simulink model "msiglabel_in"  (Simulink 6.3)
settings: Solver=FixedStepDiscrete  StartTime=0.0  StopTime=10.0  RelTol=1e-3
settings Model: Creator=awarlock  LastModifiedBy=mshakeri  ExtModeAutoUpdateStatusClock=off  StrictBusMsg=ErrorLevel1
settings OptimizationCC: InlineParams=on  InlineInvariantSignals=on
settings DebuggingCC: CheckExecutionContextPreStartOutputMsg=on  CheckExecutionContextRuntimeOutputMsg=on  SolverPrmCheckMsg=none  UnconnectedInputMsg=none  UnconnectedOutputMsg=none  UnconnectedLineMsg=none

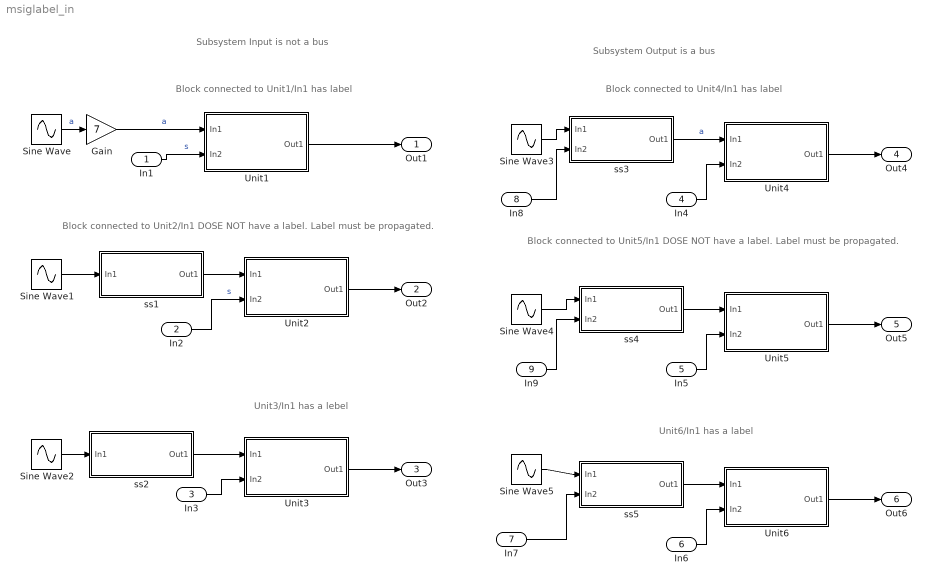
== system msiglabel_in ==
  note: Block connected to Unit1/In1 has label
  note: Block connected to Unit2/In1 DOSE NOT have a label.
      | Label must be propagated.
  note: Unit3/In1 has a lebel
  note: Subsystem Input is not a bus
  note: Subsystem Output is a bus
  note: Block connected to Unit4/In1 has label
  note: Block connected to Unit5/In1  DOSE NOT have a label.
      | Label must be propagated.
  note: Unit6/In1 has a label
  In1 : Inport  Port=1  LatchInput=off
  In2 : Inport  Port=2  LatchInput=off
  In3 : Inport  Port=3  LatchInput=off
  In4 : Inport  Port=4  LatchInput=off
  In5 : Inport  Port=5  LatchInput=off
  In6 : Inport  Port=6  LatchInput=off
  In7 : Inport  Port=7  LatchInput=off
  In8 : Inport  Port=8  LatchInput=off
  In9 : Inport  Port=9  LatchInput=off
  Gain : Gain  Gain=7
  Sine Wave{,1..5} (6 alike) : Sin  SampleTime=0
  Unit1 : Subsystem  TreatAsAtomicUnit=on
  Unit2 : Subsystem  TreatAsAtomicUnit=on
  Unit3 : Subsystem  TreatAsAtomicUnit=on
  Unit4 : Subsystem  TreatAsAtomicUnit=on
  Unit5 : Subsystem  TreatAsAtomicUnit=on
  Unit6 : Subsystem  TreatAsAtomicUnit=on
  ss1 : Subsystem
  ss2 : Subsystem
  ss3 : Subsystem
  ss4 : Subsystem
  ss5 : Subsystem
  Out1 : Outport
  Out2 : Outport  Port=2
  Out3 : Outport  Port=3
  Out4 : Outport  Port=4
  Out5 : Outport  Port=5
  Out6 : Outport  Port=6
  wires:
  Sine Wave/1 -> Gain/1  "a"
  Sine Wave1/1 -> ss1/1(In1)
  Unit1/1(Out1) -> Out1/1
  Sine Wave2/1 -> ss2/1(In1)
  Sine Wave3/1 -> ss3/1(In1)
  In1/1 -> Unit1/2(In2)  "s"
  ss1/1(Out1) -> Unit2/1(In1)
  In2/1 -> Unit2/2(In2)  "s"
  Unit2/1(Out1) -> Out2/1
  ss2/1(Out1) -> Unit3/1(In1)
  In3/1 -> Unit3/2(In2)
  Unit3/1(Out1) -> Out3/1
  ss3/1(Out1) -> Unit4/1(In1)  "a"
  In4/1 -> Unit4/2(In2)
  Unit4/1(Out1) -> Out4/1
  Sine Wave4/1 -> ss4/1(In1)
  ss4/1(Out1) -> Unit5/1(In1)
  In5/1 -> Unit5/2(In2)
  Unit5/1(Out1) -> Out5/1
  Sine Wave5/1 -> ss5/1(In1)
  ss5/1(Out1) -> Unit6/1(In1)
  In6/1 -> Unit6/2(In2)
  Unit6/1(Out1) -> Out6/1
  Gain/1 -> Unit1/1(In1)  "a"
  In7/1 -> ss5/2(In2)
  In8/1 -> ss3/2(In2)
  In9/1 -> ss4/2(In2)

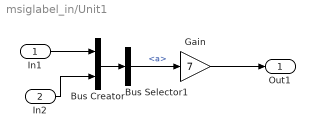
== system msiglabel_in/Unit1 ==
  In1 : Inport  Port=1  LatchInput=off
  In2 : Inport  Port=2  LatchInput=off
  Bus Creator : BusCreator  Inputs=2
  Bus Selector1 : BusSelector  OutputSignals=a
  Gain : Gain  Gain=7
  Out1 : Outport
  wires:
  Bus Creator/1 -> Bus Selector1/1
  In2/1 -> Bus Creator/2
  In1/1 -> Bus Creator/1
  Bus Selector1/1 -> Gain/1  "<a>"
  Gain/1 -> Out1/1

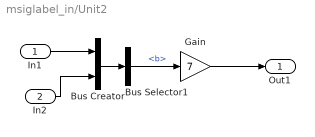
== system msiglabel_in/Unit2 ==
  In1 : Inport  Port=1  LatchInput=off
  In2 : Inport  Port=2  LatchInput=off
  Bus Creator : BusCreator  Inputs=2
  Bus Selector1 : BusSelector  OutputSignals=b
  Gain : Gain  Gain=7
  Out1 : Outport
  wires:
  Gain/1 -> Out1/1
  Bus Selector1/1 -> Gain/1  "<b>"
  In1/1 -> Bus Creator/1
  In2/1 -> Bus Creator/2
  Bus Creator/1 -> Bus Selector1/1

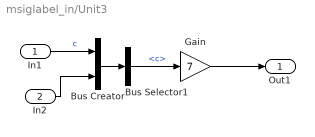
== system msiglabel_in/Unit3 ==
  In1 : Inport  Port=1  LatchInput=off
  In2 : Inport  Port=2  LatchInput=off
  Bus Creator : BusCreator  Inputs=2
  Bus Selector1 : BusSelector  OutputSignals=c
  Gain : Gain  Gain=7
  Out1 : Outport
  wires:
  Bus Creator/1 -> Bus Selector1/1
  In2/1 -> Bus Creator/2
  In1/1 -> Bus Creator/1  "c"
  Bus Selector1/1 -> Gain/1  "<c>"
  Gain/1 -> Out1/1

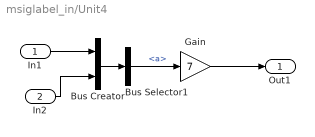
== system msiglabel_in/Unit4 ==
  In1 : Inport  Port=1  LatchInput=off
  In2 : Inport  Port=2  LatchInput=off
  Bus Creator : BusCreator  Inputs=2
  Bus Selector1 : BusSelector  OutputSignals=a
  Gain : Gain  Gain=7
  Out1 : Outport
  wires:
  Gain/1 -> Out1/1
  Bus Selector1/1 -> Gain/1  "<a>"
  In1/1 -> Bus Creator/1
  In2/1 -> Bus Creator/2
  Bus Creator/1 -> Bus Selector1/1

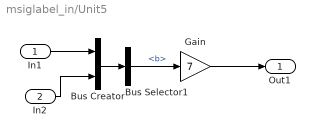
== system msiglabel_in/Unit5 ==
  In1 : Inport  Port=1  LatchInput=off
  In2 : Inport  Port=2  LatchInput=off
  Bus Creator : BusCreator  Inputs=2
  Bus Selector1 : BusSelector  OutputSignals=b
  Gain : Gain  Gain=7
  Out1 : Outport
  wires:
  Bus Creator/1 -> Bus Selector1/1
  In2/1 -> Bus Creator/2
  In1/1 -> Bus Creator/1
  Bus Selector1/1 -> Gain/1  "<b>"
  Gain/1 -> Out1/1

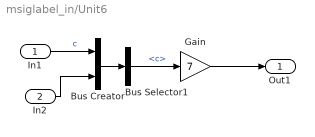
== system msiglabel_in/Unit6 ==
  In1 : Inport  Port=1  LatchInput=off
  In2 : Inport  Port=2  LatchInput=off
  Bus Creator : BusCreator  Inputs=2
  Bus Selector1 : BusSelector  OutputSignals=c
  Gain : Gain  Gain=7
  Out1 : Outport
  wires:
  Gain/1 -> Out1/1
  Bus Selector1/1 -> Gain/1  "<c>"
  In1/1 -> Bus Creator/1  "c"
  In2/1 -> Bus Creator/2
  Bus Creator/1 -> Bus Selector1/1

== system msiglabel_in/ss1 ==
  In1 : Inport  Port=1  LatchInput=off
  Subsystem : Subsystem
  Out1 : Outport
  wires:
  Subsystem/1(Out1) -> Out1/1
  In1/1 -> Subsystem/1(In1)

== system msiglabel_in/ss2 ==
  In1 : Inport  Port=1  LatchInput=off
  Subsystem : Subsystem
  Out1 : Outport
  wires:
  In1/1 -> Subsystem/1(In1)
  Subsystem/1(Out1) -> Out1/1

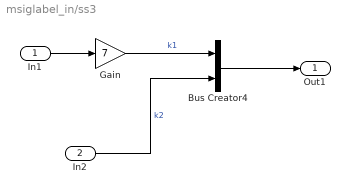
== system msiglabel_in/ss3 ==
  In1 : Inport  Port=1  LatchInput=off
  In2 : Inport  Port=2  LatchInput=off
  Bus Creator4 : BusCreator  Inputs=2
  Gain : Gain  Gain=7
  Out1 : Outport
  wires:
  In1/1 -> Gain/1
  Bus Creator4/1 -> Out1/1
  Gain/1 -> Bus Creator4/1  "k1"
  In2/1 -> Bus Creator4/2  "k2"

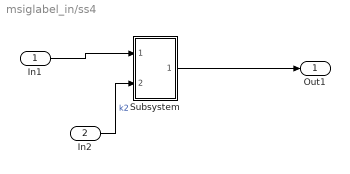
== system msiglabel_in/ss4 ==
  In1 : Inport  Port=1  LatchInput=off
  In2 : Inport  Port=2  LatchInput=off
  Subsystem : Subsystem
  Out1 : Outport
  wires:
  In2/1 -> Subsystem/2(In2)  "k2"
  Subsystem/1(Out1) -> Out1/1
  In1/1 -> Subsystem/1(In1)

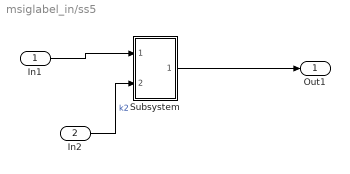
== system msiglabel_in/ss5 ==
  In1 : Inport  Port=1  LatchInput=off
  In2 : Inport  Port=2  LatchInput=off
  Subsystem : Subsystem
  Out1 : Outport
  wires:
  In1/1 -> Subsystem/1(In1)
  Subsystem/1(Out1) -> Out1/1
  In2/1 -> Subsystem/2(In2)  "k2"

== system msiglabel_in/ss1/Subsystem ==
  In1 : Inport  Port=1  LatchInput=off
  Gain : Gain  Gain=7
  Out1 : Outport
  wires:
  In1/1 -> Gain/1  "b"
  Gain/1 -> Out1/1  "b"

== system msiglabel_in/ss2/Subsystem ==
  In1 : Inport  Port=1  LatchInput=off
  Gain : Gain  Gain=7
  Out1 : Outport
  wires:
  In1/1 -> Gain/1  "d"
  Gain/1 -> Out1/1  "d"

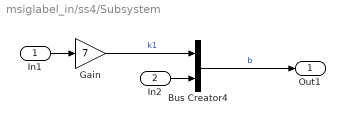
== system msiglabel_in/ss4/Subsystem ==
  In1 : Inport  Port=1  LatchInput=off
  In2 : Inport  Port=2  LatchInput=off
  Bus Creator4 : BusCreator  Inputs=2
  Gain : Gain  Gain=7
  Out1 : Outport
  wires:
  Gain/1 -> Bus Creator4/1  "k1"
  In1/1 -> Gain/1
  Bus Creator4/1 -> Out1/1  "b"
  In2/1 -> Bus Creator4/2

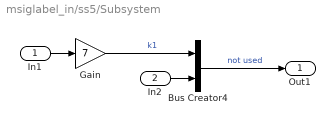
== system msiglabel_in/ss5/Subsystem ==
  In1 : Inport  Port=1  LatchInput=off
  In2 : Inport  Port=2  LatchInput=off
  Bus Creator4 : BusCreator  Inputs=2
  Gain : Gain  Gain=7
  Out1 : Outport
  wires:
  In2/1 -> Bus Creator4/2
  Bus Creator4/1 -> Out1/1  "not used"
  In1/1 -> Gain/1
  Gain/1 -> Bus Creator4/1  "k1"
